simulink model "Fan_on_off_with_if_statement"  (R2016b)
settings: Solver=VariableStepAuto  StartTime=0.0  StopTime=10.0  RelTol=1e-3
settings Model: Creator=Saher Ghanem  LastModifiedBy=Saher Ghanem

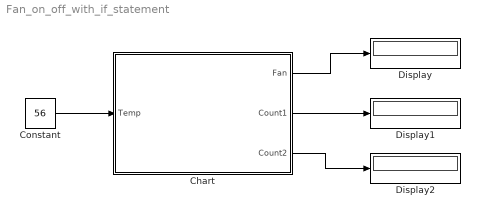
== system Fan_on_off_with_if_statement ==
  Chart : Stateflow chart  TreatAsAtomicUnit=on
  Constant : Constant  Value=56
  Display : Display
  Display1 : Display
  Display2 : Display
  wires:
  Constant/1 -> Chart/1(Temp)
  Chart/1(Fan) -> Display/1
  Chart/2(Count1) -> Display1/1
  Chart/3(Count2) -> Display2/1

== stateflow chart Fan_on_off_with_if_statement/Chart ==
  (default) -> (junction 17) : /* IF */
  (junction 17) -> (junction 18) [order 1] : [Temp>=50]
  (junction 17) -> (junction 19) [order 2] : {Fan=0;}
  (junction 18) -> (junction 20) : {Fan=1;}
  (junction 20) -> (junction 19)
  (junction 19) -> (junction 21)
  data: Temp input double; Fan output double; Count1 output double; Count2 output double
